simulink model "recordEEG"  (R2019a)
settings: Solver=VariableStepAuto  StartTime=0.0  StopTime=inf  RelTol=1e-3
undefined symbols (not defined in the file or in its folder): daq
libraries: commrandsrc3 x2, daqlib x1, dspnetwork x1
settings Model: Creator=Kusunoki  LastModifiedBy=Owner

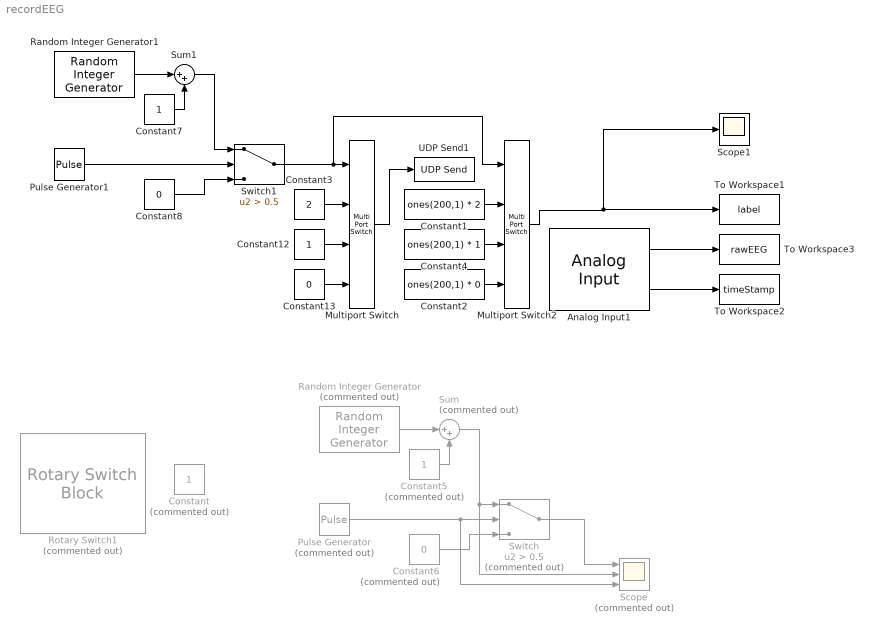
== system recordEEG ==
  Analog Input1 : daqlib/Analog Input  DeviceMenu=ni Dev1 (USB-6000)  Device=ni Dev1 (USB-6000)  ObjConstructor=daq.createSession('ni')  NChannelsSelected=3  Channels=1$ai0$$Dev1$1$1$1$1$#1$ai1$$Dev1$1$1$1$1$#1$ai2$$Dev1$1$1$1$1$#0$ai3$$Dev1$1$1$1$1$#0$ai4$$Dev1$1$1$1$1$#0$ai5$$Dev1$1$1$1$1$#0$ai6$$Dev1$1$1$1$1$#0$ai7$$Dev1$1$1$1$1$#  NPorts=1 for all channels  SampleRate=2000  ActualRate=2000.5001  ScansPerTrigger=200  OutputTimestamp=on  AcqMode=0  NumFrameBuffer=100  OutputTriggertime=off
      settings: SourceProductName=Data Acquisition Toolbox  SourceProductBaseCode=DA
  Constant : Constant  Commented=on
  Constant1 : Constant  Value=ones(200,1) * 2
  Constant12 : Constant
  Constant13 : Constant  Value=0
  Constant2 : Constant  Value=ones(200,1) * 0
  Constant3 : Constant  Value=2
  Constant4 : Constant  Value=ones(200,1) * 1
  Constant5 : Constant  Commented=on
  Constant6 : Constant  Commented=on  Value=0
  Constant7 : Constant
  Constant8 : Constant  Value=0
  Multiport Switch : MultiPortSwitch  DataPortOrder=Specify indices  DataPortIndices={2,1,0}
  Multiport Switch2 : MultiPortSwitch  DataPortOrder=Specify indices  DataPortIndices={2,1,0}
  Pulse Generator : DiscretePulseGenerator  Commented=on  PulseType=Time based  Period=12  PulseWidth=10/12 * 100
  Pulse Generator1 : DiscretePulseGenerator  PulseType=Time based  Period=13  PulseWidth=10/13 * 100
  Random Integer Generator : commrandsrc3/Random Integer Generator  Commented=on  SetSize=2  SeedSource=Auto  Seed=0  SampleTime=12  SamplesPerFrame=1  OutputDataType=uint32  SimulateUsing=Interpreted execution
      settings: SourceProductName=Communications Toolbox
  Random Integer Generator1 : commrandsrc3/Random Integer Generator  SetSize=2  SeedSource=Auto  Seed=0  SampleTime=13  SamplesPerFrame=1  OutputDataType=uint32  SimulateUsing=Interpreted execution
      settings: SourceProductName=Communications Toolbox
  Rotary Switch1 : RotarySwitchBlock  Commented=on
      settings: Values={{'0 : Relaxing', '1 : Gripping', '2 : Picking'}, [0 1 2]}
  Scope : Scope  Commented=on  NumInputPorts=3
  Scope1 : Scope
  Sum : Sum  Commented=on  Inputs=|++
  Sum1 : Sum  Inputs=|++
  Switch : Switch  Commented=on  Criteria=u2 > Threshold  Threshold=0.5
  Switch1 : Switch  Criteria=u2 > Threshold  Threshold=0.5
  To Workspace1 : ToWorkspace  VariableName=label  SampleTime=-1
  To Workspace2 : ToWorkspace  VariableName=timeStamp  SampleTime=-1
  To Workspace3 : ToWorkspace  VariableName=rawEEG  SampleTime=-1
  UDP Send1 : dspnetwork/UDP Send  remoteURL='127.0.0.1'  remotePort=25000  localURL='0.0.0.0'  localPortSource=Automatically determine  localPort=-1  sampletime=-1  blockPlatform=[]  separateLengthPort=0
      settings: SourceProductName=Simulink
  wires:
  Switch1/1 -> Multiport Switch2/1, Multiport Switch/1
  Constant12/1 -> Multiport Switch/3
  Multiport Switch/1 -> UDP Send1/1
  Analog Input1/2 -> To Workspace2/1
  Constant3/1 -> Multiport Switch/2
  Constant13/1 -> Multiport Switch/4
  Multiport Switch2/1 -> To Workspace1/1, Scope1/1
  Analog Input1/1 -> To Workspace3/1
  Constant2/1 -> Multiport Switch2/4
  Constant4/1 -> Multiport Switch2/3
  Constant1/1 -> Multiport Switch2/2
  Random Integer Generator/1 -> Sum/1
  Constant5/1 -> Sum/2
  Pulse Generator/1 -> Scope/3, Switch/2
  Constant6/1 -> Switch/3
  Switch/1 -> Scope/1
  Sum/1 -> Scope/2, Switch/1
  Sum1/1 -> Switch1/1
  Pulse Generator1/1 -> Switch1/2
  Constant7/1 -> Sum1/2
  Random Integer Generator1/1 -> Sum1/1
  Constant8/1 -> Switch1/3
